simulink model "UberSpurs"  (R2015b)
settings: Solver=VariableStepAuto  StartTime=0.0  StopTime=10000  RelTol=1e-3
(part 2 of 4)

== system UberSpurs/spur1WorkCell/route2Channel12 ==
  serverAvailable : Inport
  Constant : Constant  Value=12
  Get Attribute : GetAttribute  AttributeName=Channel  EvaluatedDefaultAttributeValue={ []}
      settings: OutputPortMap=o1
  RoutingControlBehavior : Stateflow chart  TreatAsAtomicUnit=on
  Single Server1 : SingleServer  ServiceTime=0
  route2Channel1 : OutputSwitch  NumberOutputPorts=2  SwitchingCriterion=From signal port p  InitialConditionsOpt=on
  toChannel : PMIOPort  Port=1  Side=Right
  fromMHS : PMIOPort  Port=2  Side=Left
  toMHS : PMIOPort  Port=3  Side=Right
  wires:
  RoutingControlBehavior/1(route) -> route2Channel1/1
  Constant/1 -> RoutingControlBehavior/2(channel)
  Get Attribute/1 -> RoutingControlBehavior/1(entityChannel)
  serverAvailable/1 -> RoutingControlBehavior/3(serverAvailable)
  connections:
  route2Channel1/RConn2 -- toMHS/RConn1
  Get Attribute/RConn1 -- Single Server1/LConn1
  fromMHS/RConn1 -- Get Attribute/LConn1
  toChannel/RConn1 -- route2Channel1/RConn1
  Single Server1/RConn1 -- route2Channel1/LConn1

== system UberSpurs/spur1WorkCell/route2Channel13 ==
  serverAvailable : Inport
  Constant : Constant  Value=13
  Get Attribute : GetAttribute  AttributeName=Channel  EvaluatedDefaultAttributeValue={ []}
      settings: OutputPortMap=o1
  RoutingControlBehavior : Stateflow chart  TreatAsAtomicUnit=on
  Single Server1 : SingleServer  ServiceTime=0
  route2Channel1 : OutputSwitch  NumberOutputPorts=2  SwitchingCriterion=From signal port p  InitialConditionsOpt=on
  toChannel : PMIOPort  Port=1  Side=Right
  fromMHS : PMIOPort  Port=2  Side=Left
  toMHS : PMIOPort  Port=3  Side=Right
  wires:
  RoutingControlBehavior/1(route) -> route2Channel1/1
  Constant/1 -> RoutingControlBehavior/2(channel)
  Get Attribute/1 -> RoutingControlBehavior/1(entityChannel)
  serverAvailable/1 -> RoutingControlBehavior/3(serverAvailable)
  connections:
  route2Channel1/RConn2 -- toMHS/RConn1
  Get Attribute/RConn1 -- Single Server1/LConn1
  fromMHS/RConn1 -- Get Attribute/LConn1
  toChannel/RConn1 -- route2Channel1/RConn1
  Single Server1/RConn1 -- route2Channel1/LConn1

== system UberSpurs/spur1WorkCell/route2Channel14 ==
  serverAvailable : Inport
  Constant : Constant  Value=14
  Get Attribute : GetAttribute  AttributeName=Channel  EvaluatedDefaultAttributeValue={ []}
      settings: OutputPortMap=o1
  RoutingControlBehavior : Stateflow chart  TreatAsAtomicUnit=on
  Single Server1 : SingleServer  ServiceTime=0
  route2Channel1 : OutputSwitch  NumberOutputPorts=2  SwitchingCriterion=From signal port p  InitialConditionsOpt=on
  toChannel : PMIOPort  Port=1  Side=Right
  fromMHS : PMIOPort  Port=2  Side=Left
  toMHS : PMIOPort  Port=3  Side=Right
  wires:
  RoutingControlBehavior/1(route) -> route2Channel1/1
  Constant/1 -> RoutingControlBehavior/2(channel)
  Get Attribute/1 -> RoutingControlBehavior/1(entityChannel)
  serverAvailable/1 -> RoutingControlBehavior/3(serverAvailable)
  connections:
  route2Channel1/RConn2 -- toMHS/RConn1
  Get Attribute/RConn1 -- Single Server1/LConn1
  fromMHS/RConn1 -- Get Attribute/LConn1
  toChannel/RConn1 -- route2Channel1/RConn1
  Single Server1/RConn1 -- route2Channel1/LConn1

== system UberSpurs/spur1WorkCell/route2Channel15 ==
  serverAvailable : Inport
  Constant : Constant  Value=15
  Get Attribute : GetAttribute  AttributeName=Channel  EvaluatedDefaultAttributeValue={ []}
      settings: OutputPortMap=o1
  RoutingControlBehavior : Stateflow chart  TreatAsAtomicUnit=on
  Single Server1 : SingleServer  ServiceTime=0
  route2Channel1 : OutputSwitch  NumberOutputPorts=2  SwitchingCriterion=From signal port p  InitialConditionsOpt=on
  toChannel : PMIOPort  Port=1  Side=Right
  fromMHS : PMIOPort  Port=2  Side=Left
  toMHS : PMIOPort  Port=3  Side=Right
  wires:
  RoutingControlBehavior/1(route) -> route2Channel1/1
  Constant/1 -> RoutingControlBehavior/2(channel)
  Get Attribute/1 -> RoutingControlBehavior/1(entityChannel)
  serverAvailable/1 -> RoutingControlBehavior/3(serverAvailable)
  connections:
  route2Channel1/RConn2 -- toMHS/RConn1
  Get Attribute/RConn1 -- Single Server1/LConn1
  fromMHS/RConn1 -- Get Attribute/LConn1
  toChannel/RConn1 -- route2Channel1/RConn1
  Single Server1/RConn1 -- route2Channel1/LConn1

== system UberSpurs/spur1WorkCell/route2Channel16 ==
  serverAvailable : Inport
  Constant : Constant  Value=16
  Get Attribute : GetAttribute  AttributeName=Channel  EvaluatedDefaultAttributeValue={ []}
      settings: OutputPortMap=o1
  RoutingControlBehavior : Stateflow chart  TreatAsAtomicUnit=on
  Single Server1 : SingleServer  ServiceTime=0
  route2Channel1 : OutputSwitch  NumberOutputPorts=2  SwitchingCriterion=From signal port p  InitialConditionsOpt=on
  toChannel : PMIOPort  Port=1  Side=Right
  fromMHS : PMIOPort  Port=2  Side=Left
  toMHS : PMIOPort  Port=3  Side=Right
  wires:
  RoutingControlBehavior/1(route) -> route2Channel1/1
  Constant/1 -> RoutingControlBehavior/2(channel)
  Get Attribute/1 -> RoutingControlBehavior/1(entityChannel)
  serverAvailable/1 -> RoutingControlBehavior/3(serverAvailable)
  connections:
  route2Channel1/RConn2 -- toMHS/RConn1
  Get Attribute/RConn1 -- Single Server1/LConn1
  fromMHS/RConn1 -- Get Attribute/LConn1
  toChannel/RConn1 -- route2Channel1/RConn1
  Single Server1/RConn1 -- route2Channel1/LConn1

== system UberSpurs/spur1WorkCell/route2Channel17 ==
  serverAvailable : Inport
  Constant : Constant  Value=17
  Get Attribute : GetAttribute  AttributeName=Channel  EvaluatedDefaultAttributeValue={ []}
      settings: OutputPortMap=o1
  RoutingControlBehavior : Stateflow chart  TreatAsAtomicUnit=on
  Single Server1 : SingleServer  ServiceTime=0
  route2Channel1 : OutputSwitch  NumberOutputPorts=2  SwitchingCriterion=From signal port p  InitialConditionsOpt=on
  toChannel : PMIOPort  Port=1  Side=Right
  fromMHS : PMIOPort  Port=2  Side=Left
  toMHS : PMIOPort  Port=3  Side=Right
  wires:
  RoutingControlBehavior/1(route) -> route2Channel1/1
  Constant/1 -> RoutingControlBehavior/2(channel)
  Get Attribute/1 -> RoutingControlBehavior/1(entityChannel)
  serverAvailable/1 -> RoutingControlBehavior/3(serverAvailable)
  connections:
  route2Channel1/RConn2 -- toMHS/RConn1
  Get Attribute/RConn1 -- Single Server1/LConn1
  fromMHS/RConn1 -- Get Attribute/LConn1
  toChannel/RConn1 -- route2Channel1/RConn1
  Single Server1/RConn1 -- route2Channel1/LConn1

== system UberSpurs/spur1WorkCell/route2Channel18 ==
  serverAvailable : Inport
  Constant : Constant  Value=18
  Get Attribute : GetAttribute  AttributeName=Channel  EvaluatedDefaultAttributeValue={ []}
      settings: OutputPortMap=o1
  RoutingControlBehavior : Stateflow chart  TreatAsAtomicUnit=on
  Single Server1 : SingleServer  ServiceTime=0
  route2Channel1 : OutputSwitch  NumberOutputPorts=2  SwitchingCriterion=From signal port p  InitialConditionsOpt=on
  toChannel : PMIOPort  Port=1  Side=Right
  fromMHS : PMIOPort  Port=2  Side=Left
  toMHS : PMIOPort  Port=3  Side=Right
  wires:
  RoutingControlBehavior/1(route) -> route2Channel1/1
  Constant/1 -> RoutingControlBehavior/2(channel)
  Get Attribute/1 -> RoutingControlBehavior/1(entityChannel)
  serverAvailable/1 -> RoutingControlBehavior/3(serverAvailable)
  connections:
  route2Channel1/RConn2 -- toMHS/RConn1
  Get Attribute/RConn1 -- Single Server1/LConn1
  fromMHS/RConn1 -- Get Attribute/LConn1
  toChannel/RConn1 -- route2Channel1/RConn1
  Single Server1/RConn1 -- route2Channel1/LConn1

== system UberSpurs/spur1WorkCell/route2Channel2 ==
  serverAvailable : Inport
  Constant : Constant  Value=2
  Get Attribute : GetAttribute  AttributeName=Channel  EvaluatedDefaultAttributeValue={ []}
      settings: OutputPortMap=o1
  RoutingControlBehavior : Stateflow chart  TreatAsAtomicUnit=on
  Single Server1 : SingleServer  ServiceTime=0
  route2Channel1 : OutputSwitch  NumberOutputPorts=2  SwitchingCriterion=From signal port p  InitialConditionsOpt=on
  toChannel : PMIOPort  Port=1  Side=Right
  fromMHS : PMIOPort  Port=2  Side=Left
  toMHS : PMIOPort  Port=3  Side=Right
  wires:
  RoutingControlBehavior/1(route) -> route2Channel1/1
  Constant/1 -> RoutingControlBehavior/2(channel)
  Get Attribute/1 -> RoutingControlBehavior/1(entityChannel)
  serverAvailable/1 -> RoutingControlBehavior/3(serverAvailable)
  connections:
  route2Channel1/RConn2 -- toMHS/RConn1
  Get Attribute/RConn1 -- Single Server1/LConn1
  fromMHS/RConn1 -- Get Attribute/LConn1
  toChannel/RConn1 -- route2Channel1/RConn1
  Single Server1/RConn1 -- route2Channel1/LConn1

== system UberSpurs/spur1WorkCell/route2Channel3 ==
  serverAvailable : Inport
  Constant : Constant  Value=3
  Get Attribute : GetAttribute  AttributeName=Channel  EvaluatedDefaultAttributeValue={ []}
      settings: OutputPortMap=o1
  RoutingControlBehavior : Stateflow chart  TreatAsAtomicUnit=on
  Single Server1 : SingleServer  ServiceTime=0
  route2Channel1 : OutputSwitch  NumberOutputPorts=2  SwitchingCriterion=From signal port p  InitialConditionsOpt=on
  toChannel : PMIOPort  Port=1  Side=Right
  fromMHS : PMIOPort  Port=2  Side=Left
  toMHS : PMIOPort  Port=3  Side=Right
  wires:
  RoutingControlBehavior/1(route) -> route2Channel1/1
  Constant/1 -> RoutingControlBehavior/2(channel)
  Get Attribute/1 -> RoutingControlBehavior/1(entityChannel)
  serverAvailable/1 -> RoutingControlBehavior/3(serverAvailable)
  connections:
  route2Channel1/RConn2 -- toMHS/RConn1
  Get Attribute/RConn1 -- Single Server1/LConn1
  fromMHS/RConn1 -- Get Attribute/LConn1
  toChannel/RConn1 -- route2Channel1/RConn1
  Single Server1/RConn1 -- route2Channel1/LConn1

== system UberSpurs/spur1WorkCell/route2Channel4 ==
  serverAvailable : Inport
  Constant : Constant  Value=4
  Get Attribute : GetAttribute  AttributeName=Channel  EvaluatedDefaultAttributeValue={ []}
      settings: OutputPortMap=o1
  RoutingControlBehavior : Stateflow chart  TreatAsAtomicUnit=on
  Single Server1 : SingleServer  ServiceTime=0
  route2Channel1 : OutputSwitch  NumberOutputPorts=2  SwitchingCriterion=From signal port p  InitialConditionsOpt=on
  toChannel : PMIOPort  Port=1  Side=Right
  fromMHS : PMIOPort  Port=2  Side=Left
  toMHS : PMIOPort  Port=3  Side=Right
  wires:
  RoutingControlBehavior/1(route) -> route2Channel1/1
  Constant/1 -> RoutingControlBehavior/2(channel)
  Get Attribute/1 -> RoutingControlBehavior/1(entityChannel)
  serverAvailable/1 -> RoutingControlBehavior/3(serverAvailable)
  connections:
  route2Channel1/RConn2 -- toMHS/RConn1
  Get Attribute/RConn1 -- Single Server1/LConn1
  fromMHS/RConn1 -- Get Attribute/LConn1
  toChannel/RConn1 -- route2Channel1/RConn1
  Single Server1/RConn1 -- route2Channel1/LConn1

== system UberSpurs/spur1WorkCell/route2Channel5 ==
  serverAvailable : Inport
  Constant : Constant  Value=5
  Get Attribute : GetAttribute  AttributeName=Channel  EvaluatedDefaultAttributeValue={ []}
      settings: OutputPortMap=o1
  RoutingControlBehavior : Stateflow chart  TreatAsAtomicUnit=on
  Single Server1 : SingleServer  ServiceTime=0
  route2Channel1 : OutputSwitch  NumberOutputPorts=2  SwitchingCriterion=From signal port p  InitialConditionsOpt=on
  toChannel : PMIOPort  Port=1  Side=Right
  fromMHS : PMIOPort  Port=2  Side=Left
  toMHS : PMIOPort  Port=3  Side=Right
  wires:
  RoutingControlBehavior/1(route) -> route2Channel1/1
  Constant/1 -> RoutingControlBehavior/2(channel)
  Get Attribute/1 -> RoutingControlBehavior/1(entityChannel)
  serverAvailable/1 -> RoutingControlBehavior/3(serverAvailable)
  connections:
  route2Channel1/RConn2 -- toMHS/RConn1
  Get Attribute/RConn1 -- Single Server1/LConn1
  fromMHS/RConn1 -- Get Attribute/LConn1
  toChannel/RConn1 -- route2Channel1/RConn1
  Single Server1/RConn1 -- route2Channel1/LConn1

== system UberSpurs/spur1WorkCell/route2Channel6 ==
  serverAvailable : Inport
  Constant : Constant  Value=6
  Get Attribute : GetAttribute  AttributeName=Channel  EvaluatedDefaultAttributeValue={ []}
      settings: OutputPortMap=o1
  RoutingControlBehavior : Stateflow chart  TreatAsAtomicUnit=on
  Single Server1 : SingleServer  ServiceTime=0
  route2Channel1 : OutputSwitch  NumberOutputPorts=2  SwitchingCriterion=From signal port p  InitialConditionsOpt=on
  toChannel : PMIOPort  Port=1  Side=Right
  fromMHS : PMIOPort  Port=2  Side=Left
  toMHS : PMIOPort  Port=3  Side=Right
  wires:
  RoutingControlBehavior/1(route) -> route2Channel1/1
  Constant/1 -> RoutingControlBehavior/2(channel)
  Get Attribute/1 -> RoutingControlBehavior/1(entityChannel)
  serverAvailable/1 -> RoutingControlBehavior/3(serverAvailable)
  connections:
  route2Channel1/RConn2 -- toMHS/RConn1
  Get Attribute/RConn1 -- Single Server1/LConn1
  fromMHS/RConn1 -- Get Attribute/LConn1
  toChannel/RConn1 -- route2Channel1/RConn1
  Single Server1/RConn1 -- route2Channel1/LConn1

== system UberSpurs/spur1WorkCell/route2Channel7 ==
  serverAvailable : Inport
  Constant : Constant  Value=7
  Get Attribute : GetAttribute  AttributeName=Channel  EvaluatedDefaultAttributeValue={ []}
      settings: OutputPortMap=o1
  RoutingControlBehavior : Stateflow chart  TreatAsAtomicUnit=on
  Single Server1 : SingleServer  ServiceTime=0
  route2Channel1 : OutputSwitch  NumberOutputPorts=2  SwitchingCriterion=From signal port p  InitialConditionsOpt=on
  toChannel : PMIOPort  Port=1  Side=Right
  fromMHS : PMIOPort  Port=2  Side=Left
  toMHS : PMIOPort  Port=3  Side=Right
  wires:
  RoutingControlBehavior/1(route) -> route2Channel1/1
  Constant/1 -> RoutingControlBehavior/2(channel)
  Get Attribute/1 -> RoutingControlBehavior/1(entityChannel)
  serverAvailable/1 -> RoutingControlBehavior/3(serverAvailable)
  connections:
  route2Channel1/RConn2 -- toMHS/RConn1
  Get Attribute/RConn1 -- Single Server1/LConn1
  fromMHS/RConn1 -- Get Attribute/LConn1
  toChannel/RConn1 -- route2Channel1/RConn1
  Single Server1/RConn1 -- route2Channel1/LConn1

== system UberSpurs/spur1WorkCell/route2Channel8 ==
  serverAvailable : Inport
  Constant : Constant  Value=8
  Get Attribute : GetAttribute  AttributeName=Channel  EvaluatedDefaultAttributeValue={ []}
      settings: OutputPortMap=o1
  RoutingControlBehavior : Stateflow chart  TreatAsAtomicUnit=on
  Single Server1 : SingleServer  ServiceTime=0
  route2Channel1 : OutputSwitch  NumberOutputPorts=2  SwitchingCriterion=From signal port p  InitialConditionsOpt=on
  toChannel : PMIOPort  Port=1  Side=Right
  fromMHS : PMIOPort  Port=2  Side=Left
  toMHS : PMIOPort  Port=3  Side=Right
  wires:
  RoutingControlBehavior/1(route) -> route2Channel1/1
  Constant/1 -> RoutingControlBehavior/2(channel)
  Get Attribute/1 -> RoutingControlBehavior/1(entityChannel)
  serverAvailable/1 -> RoutingControlBehavior/3(serverAvailable)
  connections:
  route2Channel1/RConn2 -- toMHS/RConn1
  Get Attribute/RConn1 -- Single Server1/LConn1
  fromMHS/RConn1 -- Get Attribute/LConn1
  toChannel/RConn1 -- route2Channel1/RConn1
  Single Server1/RConn1 -- route2Channel1/LConn1

== system UberSpurs/spur1WorkCell/route2Channel9 ==
  serverAvailable : Inport
  Constant : Constant  Value=9
  Get Attribute : GetAttribute  AttributeName=Channel  EvaluatedDefaultAttributeValue={ []}
      settings: OutputPortMap=o1
  RoutingControlBehavior : Stateflow chart  TreatAsAtomicUnit=on
  Single Server1 : SingleServer  ServiceTime=0
  route2Channel1 : OutputSwitch  NumberOutputPorts=2  SwitchingCriterion=From signal port p  InitialConditionsOpt=on
  toChannel : PMIOPort  Port=1  Side=Right
  fromMHS : PMIOPort  Port=2  Side=Left
  toMHS : PMIOPort  Port=3  Side=Right
  wires:
  RoutingControlBehavior/1(route) -> route2Channel1/1
  Constant/1 -> RoutingControlBehavior/2(channel)
  Get Attribute/1 -> RoutingControlBehavior/1(entityChannel)
  serverAvailable/1 -> RoutingControlBehavior/3(serverAvailable)
  connections:
  route2Channel1/RConn2 -- toMHS/RConn1
  Get Attribute/RConn1 -- Single Server1/LConn1
  fromMHS/RConn1 -- Get Attribute/LConn1
  toChannel/RConn1 -- route2Channel1/RConn1
  Single Server1/RConn1 -- route2Channel1/LConn1

== system UberSpurs/spur1WorkCell/route2recirculate ==
  verifyQueueLength : Inport
  Chart : Stateflow chart  TreatAsAtomicUnit=on
  Get Attribute : GetAttribute  AttributeName=FillTime  EvaluatedDefaultAttributeValue={ []}
      settings: OutputPortMap=o1
  Single Server1 : SingleServer  ServiceTime=0
  route2recirculate : OutputSwitch  NumberOutputPorts=2  SwitchingCriterion=From signal port p  InitialConditionsOpt=on  StatNumberDeparted=on  StatLastDeparturePort=on
      settings: OutputPortMap=o0,o3
  recirculate : PMIOPort  Port=1  Side=Right
  fromMHS : PMIOPort  Port=2  Side=Left
  toverify : PMIOPort  Port=3  Side=Right
  wires:
  Chart/1(route) -> route2recirculate/1
  Get Attribute/1 -> Chart/1(FillTime)
  route2recirculate/1 -> ?
  route2recirculate/2 -> ?
  verifyQueueLength/1 -> Chart/2(verifyQueue)
  connections:
  Get Attribute/RConn1 -- Single Server1/LConn1
  fromMHS/RConn1 -- Get Attribute/LConn1
  Single Server1/RConn1 -- route2recirculate/LConn1
  route2recirculate/RConn2 -- toverify/RConn1
  route2recirculate/RConn1 -- recirculate/RConn1

== system UberSpurs/spur1WorkCell/verifyWorkstation ==
  Clock : Clock
  Set Attribute1 : SetAttribute  AttributeName=VerifyTime  AttributeFrom=Signal port  EvaluatedAttributeValue={ []}
  Timed to Event Sigal : TimedToEventSignal
  VerifyQueue : FIFOQueue  Capacity=12  StatNumberInBlock=on
      settings: OutputPortMap=o1
  VerifyServer : SingleServer  ServiceTimeFrom=Signal port t  ServiceTime=1.55
  processTime : EventBasedRandomNumber  Distribution=Arbitrary discrete  valueVecDisc=[0 1.55]  probVecDisc=[0 1]  Seed=19165
  vialOUT : PMIOPort  Port=1  Side=Left
  vialIN : PMIOPort  Port=2  Side=Right
  queueLength : Outport
  wires:
  processTime/1 -> VerifyServer/1
  Clock/1 -> Timed to Event Sigal/1
  Timed to Event Sigal/1 -> Set Attribute1/1
  VerifyQueue/1 -> queueLength/1
  connections:
  Set Attribute1/RConn1 -- vialOUT/RConn1
  VerifyQueue/RConn1 -- VerifyServer/LConn1
  VerifyQueue/LConn1 -- vialIN/RConn1
  Set Attribute1/LConn1 -- VerifyServer/RConn1

== system UberSpurs/spur2WorkCell/fillChannel1 ==
  Clock : Clock
  Set Attribute : SetAttribute  AttributeName=FillTime  AttributeFrom=Signal port  EvaluatedAttributeValue={ []}
  Timed to Event Signal : TimedToEventSignal
  fillQueue : FIFOQueue  Capacity=1
  fillServer : SingleServer  ServiceTimeFrom=Signal port t  ServiceTime=20  StatNumberInBlock=on
      settings: OutputPortMap=o1
  processTime : EventBasedRandomNumber  Distribution=Gaussian (normal)  meanNorm=25  stdNorm=2.5  Seed=22382
  vialIN : PMIOPort  Port=1  Side=Left
  vialOut : PMIOPort  Port=2  Side=Right
  serverAvailable : Outport
  wires:
  processTime/1 -> fillServer/1
  Clock/1 -> Timed to Event Signal/1
  Timed to Event Signal/1 -> Set Attribute/1
  fillServer/1 -> serverAvailable/1
  connections:
  fillQueue/RConn1 -- fillServer/LConn1
  fillQueue/LConn1 -- vialIN/RConn1
  fillServer/RConn1 -- Set Attribute/LConn1
  Set Attribute/RConn1 -- vialOut/RConn1

== system UberSpurs/spur2WorkCell/fillChannel10 ==
  Clock : Clock
  Set Attribute : SetAttribute  AttributeName=FillTime  AttributeFrom=Signal port  EvaluatedAttributeValue={ []}
  Timed to Event Signal : TimedToEventSignal
  fillQueue : FIFOQueue  Capacity=1
  fillServer : SingleServer  ServiceTimeFrom=Signal port t  ServiceTime=20  StatNumberInBlock=on
      settings: OutputPortMap=o1
  processTime : EventBasedRandomNumber  Distribution=Gaussian (normal)  meanNorm=25  stdNorm=2.5  Seed=25599
  vialIN : PMIOPort  Port=1  Side=Left
  vialOut : PMIOPort  Port=2  Side=Right
  serverAvailable : Outport
  wires:
  processTime/1 -> fillServer/1
  Clock/1 -> Timed to Event Signal/1
  Timed to Event Signal/1 -> Set Attribute/1
  fillServer/1 -> serverAvailable/1
  connections:
  fillQueue/RConn1 -- fillServer/LConn1
  fillQueue/LConn1 -- vialIN/RConn1
  fillServer/RConn1 -- Set Attribute/LConn1
  Set Attribute/RConn1 -- vialOut/RConn1

== system UberSpurs/spur2WorkCell/fillChannel11 ==
  Clock : Clock
  Set Attribute : SetAttribute  AttributeName=FillTime  AttributeFrom=Signal port  EvaluatedAttributeValue={ []}
  Timed to Event Signal : TimedToEventSignal
  fillQueue : FIFOQueue  Capacity=1
  fillServer : SingleServer  ServiceTimeFrom=Signal port t  ServiceTime=20  StatNumberInBlock=on
      settings: OutputPortMap=o1
  processTime : EventBasedRandomNumber  Distribution=Gaussian (normal)  meanNorm=25  stdNorm=2.5  Seed=28816
  vialIN : PMIOPort  Port=1  Side=Left
  vialOut : PMIOPort  Port=2  Side=Right
  serverAvailable : Outport
  wires:
  processTime/1 -> fillServer/1
  Clock/1 -> Timed to Event Signal/1
  Timed to Event Signal/1 -> Set Attribute/1
  fillServer/1 -> serverAvailable/1
  connections:
  fillQueue/RConn1 -- fillServer/LConn1
  fillQueue/LConn1 -- vialIN/RConn1
  fillServer/RConn1 -- Set Attribute/LConn1
  Set Attribute/RConn1 -- vialOut/RConn1

== system UberSpurs/spur2WorkCell/fillChannel12 ==
  Clock : Clock
  Set Attribute : SetAttribute  AttributeName=FillTime  AttributeFrom=Signal port  EvaluatedAttributeValue={ []}
  Timed to Event Signal : TimedToEventSignal
  fillQueue : FIFOQueue  Capacity=1
  fillServer : SingleServer  ServiceTimeFrom=Signal port t  ServiceTime=20  StatNumberInBlock=on
      settings: OutputPortMap=o1
  processTime : EventBasedRandomNumber  Distribution=Gaussian (normal)  meanNorm=25  stdNorm=2.5  Seed=32033
  vialIN : PMIOPort  Port=1  Side=Left
  vialOut : PMIOPort  Port=2  Side=Right
  serverAvailable : Outport
  wires:
  processTime/1 -> fillServer/1
  Clock/1 -> Timed to Event Signal/1
  Timed to Event Signal/1 -> Set Attribute/1
  fillServer/1 -> serverAvailable/1
  connections:
  fillQueue/RConn1 -- fillServer/LConn1
  fillQueue/LConn1 -- vialIN/RConn1
  fillServer/RConn1 -- Set Attribute/LConn1
  Set Attribute/RConn1 -- vialOut/RConn1

== system UberSpurs/spur2WorkCell/fillChannel13 ==
  Clock : Clock
  Set Attribute : SetAttribute  AttributeName=FillTime  AttributeFrom=Signal port  EvaluatedAttributeValue={ []}
  Timed to Event Signal : TimedToEventSignal
  fillQueue : FIFOQueue  Capacity=1
  fillServer : SingleServer  ServiceTimeFrom=Signal port t  ServiceTime=20  StatNumberInBlock=on
      settings: OutputPortMap=o1
  processTime : EventBasedRandomNumber  Distribution=Gaussian (normal)  meanNorm=25  stdNorm=2.5  Seed=35250
  vialIN : PMIOPort  Port=1  Side=Left
  vialOut : PMIOPort  Port=2  Side=Right
  serverAvailable : Outport
  wires:
  processTime/1 -> fillServer/1
  Clock/1 -> Timed to Event Signal/1
  Timed to Event Signal/1 -> Set Attribute/1
  fillServer/1 -> serverAvailable/1
  connections:
  fillQueue/RConn1 -- fillServer/LConn1
  fillQueue/LConn1 -- vialIN/RConn1
  fillServer/RConn1 -- Set Attribute/LConn1
  Set Attribute/RConn1 -- vialOut/RConn1

== system UberSpurs/spur2WorkCell/fillChannel14 ==
  Clock : Clock
  Set Attribute : SetAttribute  AttributeName=FillTime  AttributeFrom=Signal port  EvaluatedAttributeValue={ []}
  Timed to Event Signal : TimedToEventSignal
  fillQueue : FIFOQueue  Capacity=1
  fillServer : SingleServer  ServiceTimeFrom=Signal port t  ServiceTime=20  StatNumberInBlock=on
      settings: OutputPortMap=o1
  processTime : EventBasedRandomNumber  Distribution=Gaussian (normal)  meanNorm=25  stdNorm=2.5  Seed=38467
  vialIN : PMIOPort  Port=1  Side=Left
  vialOut : PMIOPort  Port=2  Side=Right
  serverAvailable : Outport
  wires:
  processTime/1 -> fillServer/1
  Clock/1 -> Timed to Event Signal/1
  Timed to Event Signal/1 -> Set Attribute/1
  fillServer/1 -> serverAvailable/1
  connections:
  fillQueue/RConn1 -- fillServer/LConn1
  fillQueue/LConn1 -- vialIN/RConn1
  fillServer/RConn1 -- Set Attribute/LConn1
  Set Attribute/RConn1 -- vialOut/RConn1

== system UberSpurs/spur2WorkCell/fillChannel15 ==
  Clock : Clock
  Set Attribute : SetAttribute  AttributeName=FillTime  AttributeFrom=Signal port  EvaluatedAttributeValue={ []}
  Timed to Event Signal : TimedToEventSignal
  fillQueue : FIFOQueue  Capacity=1
  fillServer : SingleServer  ServiceTimeFrom=Signal port t  ServiceTime=20  StatNumberInBlock=on
      settings: OutputPortMap=o1
  processTime : EventBasedRandomNumber  Distribution=Gaussian (normal)  meanNorm=25  stdNorm=2.5  Seed=41684
  vialIN : PMIOPort  Port=1  Side=Left
  vialOut : PMIOPort  Port=2  Side=Right
  serverAvailable : Outport
  wires:
  processTime/1 -> fillServer/1
  Clock/1 -> Timed to Event Signal/1
  Timed to Event Signal/1 -> Set Attribute/1
  fillServer/1 -> serverAvailable/1
  connections:
  fillQueue/RConn1 -- fillServer/LConn1
  fillQueue/LConn1 -- vialIN/RConn1
  fillServer/RConn1 -- Set Attribute/LConn1
  Set Attribute/RConn1 -- vialOut/RConn1

== system UberSpurs/spur2WorkCell/fillChannel16 ==
  Clock : Clock
  Set Attribute : SetAttribute  AttributeName=FillTime  AttributeFrom=Signal port  EvaluatedAttributeValue={ []}
  Timed to Event Signal : TimedToEventSignal
  fillQueue : FIFOQueue  Capacity=1
  fillServer : SingleServer  ServiceTimeFrom=Signal port t  ServiceTime=20  StatNumberInBlock=on
      settings: OutputPortMap=o1
  processTime : EventBasedRandomNumber  Distribution=Gaussian (normal)  meanNorm=25  stdNorm=2.5  Seed=44901
  vialIN : PMIOPort  Port=1  Side=Left
  vialOut : PMIOPort  Port=2  Side=Right
  serverAvailable : Outport
  wires:
  processTime/1 -> fillServer/1
  Clock/1 -> Timed to Event Signal/1
  Timed to Event Signal/1 -> Set Attribute/1
  fillServer/1 -> serverAvailable/1
  connections:
  fillQueue/RConn1 -- fillServer/LConn1
  fillQueue/LConn1 -- vialIN/RConn1
  fillServer/RConn1 -- Set Attribute/LConn1
  Set Attribute/RConn1 -- vialOut/RConn1

== system UberSpurs/spur2WorkCell/fillChannel17 ==
  Clock : Clock
  Set Attribute : SetAttribute  AttributeName=FillTime  AttributeFrom=Signal port  EvaluatedAttributeValue={ []}
  Timed to Event Signal : TimedToEventSignal
  fillQueue : FIFOQueue  Capacity=1
  fillServer : SingleServer  ServiceTimeFrom=Signal port t  ServiceTime=20  StatNumberInBlock=on
      settings: OutputPortMap=o1
  processTime : EventBasedRandomNumber  Distribution=Gaussian (normal)  meanNorm=25  stdNorm=2.5  Seed=48118
  vialIN : PMIOPort  Port=1  Side=Left
  vialOut : PMIOPort  Port=2  Side=Right
  serverAvailable : Outport
  wires:
  processTime/1 -> fillServer/1
  Clock/1 -> Timed to Event Signal/1
  Timed to Event Signal/1 -> Set Attribute/1
  fillServer/1 -> serverAvailable/1
  connections:
  fillQueue/RConn1 -- fillServer/LConn1
  fillQueue/LConn1 -- vialIN/RConn1
  fillServer/RConn1 -- Set Attribute/LConn1
  Set Attribute/RConn1 -- vialOut/RConn1

== system UberSpurs/spur2WorkCell/fillChannel18 ==
  Clock : Clock
  Set Attribute : SetAttribute  AttributeName=FillTime  AttributeFrom=Signal port  EvaluatedAttributeValue={ []}
  Timed to Event Signal : TimedToEventSignal
  fillQueue : FIFOQueue  Capacity=1
  fillServer : SingleServer  ServiceTimeFrom=Signal port t  ServiceTime=20  StatNumberInBlock=on
      settings: OutputPortMap=o1
  processTime : EventBasedRandomNumber  Distribution=Gaussian (normal)  meanNorm=25  stdNorm=2.5  Seed=51335
  vialIN : PMIOPort  Port=1  Side=Left
  vialOut : PMIOPort  Port=2  Side=Right
  serverAvailable : Outport
  wires:
  processTime/1 -> fillServer/1
  Clock/1 -> Timed to Event Signal/1
  Timed to Event Signal/1 -> Set Attribute/1
  fillServer/1 -> serverAvailable/1
  connections:
  fillQueue/RConn1 -- fillServer/LConn1
  fillQueue/LConn1 -- vialIN/RConn1
  fillServer/RConn1 -- Set Attribute/LConn1
  Set Attribute/RConn1 -- vialOut/RConn1

== system UberSpurs/spur2WorkCell/fillChannel2 ==
  Clock : Clock
  Set Attribute : SetAttribute  AttributeName=FillTime  AttributeFrom=Signal port  EvaluatedAttributeValue={ []}
  Timed to Event Signal : TimedToEventSignal
  fillQueue : FIFOQueue  Capacity=1
  fillServer : SingleServer  ServiceTimeFrom=Signal port t  ServiceTime=20  StatNumberInBlock=on
      settings: OutputPortMap=o1
  processTime : EventBasedRandomNumber  Distribution=Gaussian (normal)  meanNorm=25  stdNorm=2.5  Seed=54552
  vialIN : PMIOPort  Port=1  Side=Left
  vialOut : PMIOPort  Port=2  Side=Right
  serverAvailable : Outport
  wires:
  processTime/1 -> fillServer/1
  Clock/1 -> Timed to Event Signal/1
  Timed to Event Signal/1 -> Set Attribute/1
  fillServer/1 -> serverAvailable/1
  connections:
  fillQueue/RConn1 -- fillServer/LConn1
  fillQueue/LConn1 -- vialIN/RConn1
  fillServer/RConn1 -- Set Attribute/LConn1
  Set Attribute/RConn1 -- vialOut/RConn1

== system UberSpurs/spur2WorkCell/fillChannel3 ==
  Clock : Clock
  Set Attribute : SetAttribute  AttributeName=FillTime  AttributeFrom=Signal port  EvaluatedAttributeValue={ []}
  Timed to Event Signal : TimedToEventSignal
  fillQueue : FIFOQueue  Capacity=1
  fillServer : SingleServer  ServiceTimeFrom=Signal port t  ServiceTime=20  StatNumberInBlock=on
      settings: OutputPortMap=o1
  processTime : EventBasedRandomNumber  Distribution=Gaussian (normal)  meanNorm=25  stdNorm=2.5  Seed=57769
  vialIN : PMIOPort  Port=1  Side=Left
  vialOut : PMIOPort  Port=2  Side=Right
  serverAvailable : Outport
  wires:
  processTime/1 -> fillServer/1
  Clock/1 -> Timed to Event Signal/1
  Timed to Event Signal/1 -> Set Attribute/1
  fillServer/1 -> serverAvailable/1
  connections:
  fillQueue/RConn1 -- fillServer/LConn1
  fillQueue/LConn1 -- vialIN/RConn1
  fillServer/RConn1 -- Set Attribute/LConn1
  Set Attribute/RConn1 -- vialOut/RConn1

== system UberSpurs/spur2WorkCell/fillChannel4 ==
  Clock : Clock
  Set Attribute : SetAttribute  AttributeName=FillTime  AttributeFrom=Signal port  EvaluatedAttributeValue={ []}
  Timed to Event Signal : TimedToEventSignal
  fillQueue : FIFOQueue  Capacity=1
  fillServer : SingleServer  ServiceTimeFrom=Signal port t  ServiceTime=20  StatNumberInBlock=on
      settings: OutputPortMap=o1
  processTime : EventBasedRandomNumber  Distribution=Gaussian (normal)  meanNorm=25  stdNorm=2.5  Seed=60986
  vialIN : PMIOPort  Port=1  Side=Left
  vialOut : PMIOPort  Port=2  Side=Right
  serverAvailable : Outport
  wires:
  processTime/1 -> fillServer/1
  Clock/1 -> Timed to Event Signal/1
  Timed to Event Signal/1 -> Set Attribute/1
  fillServer/1 -> serverAvailable/1
  connections:
  fillQueue/RConn1 -- fillServer/LConn1
  fillQueue/LConn1 -- vialIN/RConn1
  fillServer/RConn1 -- Set Attribute/LConn1
  Set Attribute/RConn1 -- vialOut/RConn1

== system UberSpurs/spur2WorkCell/fillChannel5 ==
  Clock : Clock
  Set Attribute : SetAttribute  AttributeName=FillTime  AttributeFrom=Signal port  EvaluatedAttributeValue={ []}
  Timed to Event Signal : TimedToEventSignal
  fillQueue : FIFOQueue  Capacity=1
  fillServer : SingleServer  ServiceTimeFrom=Signal port t  ServiceTime=20  StatNumberInBlock=on
      settings: OutputPortMap=o1
  processTime : EventBasedRandomNumber  Distribution=Gaussian (normal)  meanNorm=25  stdNorm=2.5  Seed=64203
  vialIN : PMIOPort  Port=1  Side=Left
  vialOut : PMIOPort  Port=2  Side=Right
  serverAvailable : Outport
  wires:
  processTime/1 -> fillServer/1
  Clock/1 -> Timed to Event Signal/1
  Timed to Event Signal/1 -> Set Attribute/1
  fillServer/1 -> serverAvailable/1
  connections:
  fillQueue/RConn1 -- fillServer/LConn1
  fillQueue/LConn1 -- vialIN/RConn1
  fillServer/RConn1 -- Set Attribute/LConn1
  Set Attribute/RConn1 -- vialOut/RConn1

== system UberSpurs/spur2WorkCell/fillChannel6 ==
  Clock : Clock
  Set Attribute : SetAttribute  AttributeName=FillTime  AttributeFrom=Signal port  EvaluatedAttributeValue={ []}
  Timed to Event Signal : TimedToEventSignal
  fillQueue : FIFOQueue  Capacity=1
  fillServer : SingleServer  ServiceTimeFrom=Signal port t  ServiceTime=20  StatNumberInBlock=on
      settings: OutputPortMap=o1
  processTime : EventBasedRandomNumber  Distribution=Gaussian (normal)  meanNorm=25  stdNorm=2.5  Seed=1884
  vialIN : PMIOPort  Port=1  Side=Left
  vialOut : PMIOPort  Port=2  Side=Right
  serverAvailable : Outport
  wires:
  processTime/1 -> fillServer/1
  Clock/1 -> Timed to Event Signal/1
  Timed to Event Signal/1 -> Set Attribute/1
  fillServer/1 -> serverAvailable/1
  connections:
  fillQueue/RConn1 -- fillServer/LConn1
  fillQueue/LConn1 -- vialIN/RConn1
  fillServer/RConn1 -- Set Attribute/LConn1
  Set Attribute/RConn1 -- vialOut/RConn1

== system UberSpurs/spur2WorkCell/fillChannel7 ==
  Clock : Clock
  Set Attribute : SetAttribute  AttributeName=FillTime  AttributeFrom=Signal port  EvaluatedAttributeValue={ []}
  Timed to Event Signal : TimedToEventSignal
  fillQueue : FIFOQueue  Capacity=1
  fillServer : SingleServer  ServiceTimeFrom=Signal port t  ServiceTime=20  StatNumberInBlock=on
      settings: OutputPortMap=o1
  processTime : EventBasedRandomNumber  Distribution=Gaussian (normal)  meanNorm=25  stdNorm=2.5  Seed=5101
  vialIN : PMIOPort  Port=1  Side=Left
  vialOut : PMIOPort  Port=2  Side=Right
  serverAvailable : Outport
  wires:
  processTime/1 -> fillServer/1
  Clock/1 -> Timed to Event Signal/1
  Timed to Event Signal/1 -> Set Attribute/1
  fillServer/1 -> serverAvailable/1
  connections:
  fillQueue/RConn1 -- fillServer/LConn1
  fillQueue/LConn1 -- vialIN/RConn1
  fillServer/RConn1 -- Set Attribute/LConn1
  Set Attribute/RConn1 -- vialOut/RConn1

== system UberSpurs/spur2WorkCell/fillChannel8 ==
  Clock : Clock
  Set Attribute : SetAttribute  AttributeName=FillTime  AttributeFrom=Signal port  EvaluatedAttributeValue={ []}
  Timed to Event Signal : TimedToEventSignal
  fillQueue : FIFOQueue  Capacity=1
  fillServer : SingleServer  ServiceTimeFrom=Signal port t  ServiceTime=20  StatNumberInBlock=on
      settings: OutputPortMap=o1
  processTime : EventBasedRandomNumber  Distribution=Gaussian (normal)  meanNorm=25  stdNorm=2.5  Seed=8318
  vialIN : PMIOPort  Port=1  Side=Left
  vialOut : PMIOPort  Port=2  Side=Right
  serverAvailable : Outport
  wires:
  processTime/1 -> fillServer/1
  Clock/1 -> Timed to Event Signal/1
  Timed to Event Signal/1 -> Set Attribute/1
  fillServer/1 -> serverAvailable/1
  connections:
  fillQueue/RConn1 -- fillServer/LConn1
  fillQueue/LConn1 -- vialIN/RConn1
  fillServer/RConn1 -- Set Attribute/LConn1
  Set Attribute/RConn1 -- vialOut/RConn1

== system UberSpurs/spur2WorkCell/fillChannel9 ==
  Clock : Clock
  Set Attribute : SetAttribute  AttributeName=FillTime  AttributeFrom=Signal port  EvaluatedAttributeValue={ []}
  Timed to Event Signal : TimedToEventSignal
  fillQueue : FIFOQueue  Capacity=1
  fillServer : SingleServer  ServiceTimeFrom=Signal port t  ServiceTime=20  StatNumberInBlock=on
      settings: OutputPortMap=o1
  processTime : EventBasedRandomNumber  Distribution=Gaussian (normal)  meanNorm=25  stdNorm=2.5  Seed=11535
  vialIN : PMIOPort  Port=1  Side=Left
  vialOut : PMIOPort  Port=2  Side=Right
  serverAvailable : Outport
  wires:
  processTime/1 -> fillServer/1
  Clock/1 -> Timed to Event Signal/1
  Timed to Event Signal/1 -> Set Attribute/1
  fillServer/1 -> serverAvailable/1
  connections:
  fillQueue/RConn1 -- fillServer/LConn1
  fillQueue/LConn1 -- vialIN/RConn1
  fillServer/RConn1 -- Set Attribute/LConn1
  Set Attribute/RConn1 -- vialOut/RConn1

== system UberSpurs/spur2WorkCell/route2Channel1 ==
  serverAvailable : Inport
  Constant : Constant
  Get Attribute : GetAttribute  AttributeName=Channel  EvaluatedDefaultAttributeValue={ []}
      settings: OutputPortMap=o1
  RoutingControlActuator : OutputSwitch  NumberOutputPorts=2  SwitchingCriterion=From signal port p  InitialConditionsOpt=on
  RoutingControlBehavior : Stateflow chart  TreatAsAtomicUnit=on
  Single Server1 : SingleServer  ServiceTime=0
  toChannel : PMIOPort  Port=1  Side=Right
  fromMHS : PMIOPort  Port=2  Side=Left
  toMHS : PMIOPort  Port=3  Side=Right
  wires:
  RoutingControlBehavior/1(route) -> RoutingControlActuator/1
  Constant/1 -> RoutingControlBehavior/2(channel)
  Get Attribute/1 -> RoutingControlBehavior/1(entityChannel)
  serverAvailable/1 -> RoutingControlBehavior/3(serverAvailable)
  connections:
  RoutingControlActuator/RConn2 -- toMHS/RConn1
  Get Attribute/RConn1 -- Single Server1/LConn1
  fromMHS/RConn1 -- Get Attribute/LConn1
  toChannel/RConn1 -- RoutingControlActuator/RConn1
  Single Server1/RConn1 -- RoutingControlActuator/LConn1

== system UberSpurs/spur2WorkCell/route2Channel10 ==
  serverAvailable : Inport
  Constant : Constant  Value=10
  Get Attribute : GetAttribute  AttributeName=Channel  EvaluatedDefaultAttributeValue={ []}
      settings: OutputPortMap=o1
  RoutingControlBehavior : Stateflow chart  TreatAsAtomicUnit=on
  Single Server1 : SingleServer  ServiceTime=0
  route2Channel1 : OutputSwitch  NumberOutputPorts=2  SwitchingCriterion=From signal port p  InitialConditionsOpt=on
  toChannel : PMIOPort  Port=1  Side=Right
  fromMHS : PMIOPort  Port=2  Side=Left
  toMHS : PMIOPort  Port=3  Side=Right
  wires:
  RoutingControlBehavior/1(route) -> route2Channel1/1
  Constant/1 -> RoutingControlBehavior/2(channel)
  Get Attribute/1 -> RoutingControlBehavior/1(entityChannel)
  serverAvailable/1 -> RoutingControlBehavior/3(serverAvailable)
  connections:
  route2Channel1/RConn2 -- toMHS/RConn1
  Get Attribute/RConn1 -- Single Server1/LConn1
  fromMHS/RConn1 -- Get Attribute/LConn1
  toChannel/RConn1 -- route2Channel1/RConn1
  Single Server1/RConn1 -- route2Channel1/LConn1

== system UberSpurs/spur2WorkCell/route2Channel11 ==
  serverAvailable : Inport
  Constant : Constant  Value=11
  Get Attribute : GetAttribute  AttributeName=Channel  EvaluatedDefaultAttributeValue={ []}
      settings: OutputPortMap=o1
  RoutingControlBehavior : Stateflow chart  TreatAsAtomicUnit=on
  Single Server1 : SingleServer  ServiceTime=0
  route2Channel1 : OutputSwitch  NumberOutputPorts=2  SwitchingCriterion=From signal port p  InitialConditionsOpt=on
  toChannel : PMIOPort  Port=1  Side=Right
  fromMHS : PMIOPort  Port=2  Side=Left
  toMHS : PMIOPort  Port=3  Side=Right
  wires:
  RoutingControlBehavior/1(route) -> route2Channel1/1
  Constant/1 -> RoutingControlBehavior/2(channel)
  Get Attribute/1 -> RoutingControlBehavior/1(entityChannel)
  serverAvailable/1 -> RoutingControlBehavior/3(serverAvailable)
  connections:
  route2Channel1/RConn2 -- toMHS/RConn1
  Get Attribute/RConn1 -- Single Server1/LConn1
  fromMHS/RConn1 -- Get Attribute/LConn1
  toChannel/RConn1 -- route2Channel1/RConn1
  Single Server1/RConn1 -- route2Channel1/LConn1

== system UberSpurs/spur2WorkCell/route2Channel12 ==
  serverAvailable : Inport
  Constant : Constant  Value=12
  Get Attribute : GetAttribute  AttributeName=Channel  EvaluatedDefaultAttributeValue={ []}
      settings: OutputPortMap=o1
  RoutingControlBehavior : Stateflow chart  TreatAsAtomicUnit=on
  Single Server1 : SingleServer  ServiceTime=0
  route2Channel1 : OutputSwitch  NumberOutputPorts=2  SwitchingCriterion=From signal port p  InitialConditionsOpt=on
  toChannel : PMIOPort  Port=1  Side=Right
  fromMHS : PMIOPort  Port=2  Side=Left
  toMHS : PMIOPort  Port=3  Side=Right
  wires:
  RoutingControlBehavior/1(route) -> route2Channel1/1
  Constant/1 -> RoutingControlBehavior/2(channel)
  Get Attribute/1 -> RoutingControlBehavior/1(entityChannel)
  serverAvailable/1 -> RoutingControlBehavior/3(serverAvailable)
  connections:
  route2Channel1/RConn2 -- toMHS/RConn1
  Get Attribute/RConn1 -- Single Server1/LConn1
  fromMHS/RConn1 -- Get Attribute/LConn1
  toChannel/RConn1 -- route2Channel1/RConn1
  Single Server1/RConn1 -- route2Channel1/LConn1

== system UberSpurs/spur2WorkCell/route2Channel13 ==
  serverAvailable : Inport
  Constant : Constant  Value=13
  Get Attribute : GetAttribute  AttributeName=Channel  EvaluatedDefaultAttributeValue={ []}
      settings: OutputPortMap=o1
  RoutingControlBehavior : Stateflow chart  TreatAsAtomicUnit=on
  Single Server1 : SingleServer  ServiceTime=0
  route2Channel1 : OutputSwitch  NumberOutputPorts=2  SwitchingCriterion=From signal port p  InitialConditionsOpt=on
  toChannel : PMIOPort  Port=1  Side=Right
  fromMHS : PMIOPort  Port=2  Side=Left
  toMHS : PMIOPort  Port=3  Side=Right
  wires:
  RoutingControlBehavior/1(route) -> route2Channel1/1
  Constant/1 -> RoutingControlBehavior/2(channel)
  Get Attribute/1 -> RoutingControlBehavior/1(entityChannel)
  serverAvailable/1 -> RoutingControlBehavior/3(serverAvailable)
  connections:
  route2Channel1/RConn2 -- toMHS/RConn1
  Get Attribute/RConn1 -- Single Server1/LConn1
  fromMHS/RConn1 -- Get Attribute/LConn1
  toChannel/RConn1 -- route2Channel1/RConn1
  Single Server1/RConn1 -- route2Channel1/LConn1

== system UberSpurs/spur2WorkCell/route2Channel14 ==
  serverAvailable : Inport
  Constant : Constant  Value=14
  Get Attribute : GetAttribute  AttributeName=Channel  EvaluatedDefaultAttributeValue={ []}
      settings: OutputPortMap=o1
  RoutingControlBehavior : Stateflow chart  TreatAsAtomicUnit=on
  Single Server1 : SingleServer  ServiceTime=0
  route2Channel1 : OutputSwitch  NumberOutputPorts=2  SwitchingCriterion=From signal port p  InitialConditionsOpt=on
  toChannel : PMIOPort  Port=1  Side=Right
  fromMHS : PMIOPort  Port=2  Side=Left
  toMHS : PMIOPort  Port=3  Side=Right
  wires:
  RoutingControlBehavior/1(route) -> route2Channel1/1
  Constant/1 -> RoutingControlBehavior/2(channel)
  Get Attribute/1 -> RoutingControlBehavior/1(entityChannel)
  serverAvailable/1 -> RoutingControlBehavior/3(serverAvailable)
  connections:
  route2Channel1/RConn2 -- toMHS/RConn1
  Get Attribute/RConn1 -- Single Server1/LConn1
  fromMHS/RConn1 -- Get Attribute/LConn1
  toChannel/RConn1 -- route2Channel1/RConn1
  Single Server1/RConn1 -- route2Channel1/LConn1

== system UberSpurs/spur2WorkCell/route2Channel15 ==
  serverAvailable : Inport
  Constant : Constant  Value=15
  Get Attribute : GetAttribute  AttributeName=Channel  EvaluatedDefaultAttributeValue={ []}
      settings: OutputPortMap=o1
  RoutingControlBehavior : Stateflow chart  TreatAsAtomicUnit=on
  Single Server1 : SingleServer  ServiceTime=0
  route2Channel1 : OutputSwitch  NumberOutputPorts=2  SwitchingCriterion=From signal port p  InitialConditionsOpt=on
  toChannel : PMIOPort  Port=1  Side=Right
  fromMHS : PMIOPort  Port=2  Side=Left
  toMHS : PMIOPort  Port=3  Side=Right
  wires:
  RoutingControlBehavior/1(route) -> route2Channel1/1
  Constant/1 -> RoutingControlBehavior/2(channel)
  Get Attribute/1 -> RoutingControlBehavior/1(entityChannel)
  serverAvailable/1 -> RoutingControlBehavior/3(serverAvailable)
  connections:
  route2Channel1/RConn2 -- toMHS/RConn1
  Get Attribute/RConn1 -- Single Server1/LConn1
  fromMHS/RConn1 -- Get Attribute/LConn1
  toChannel/RConn1 -- route2Channel1/RConn1
  Single Server1/RConn1 -- route2Channel1/LConn1

== system UberSpurs/spur2WorkCell/route2Channel16 ==
  serverAvailable : Inport
  Constant : Constant  Value=16
  Get Attribute : GetAttribute  AttributeName=Channel  EvaluatedDefaultAttributeValue={ []}
      settings: OutputPortMap=o1
  RoutingControlBehavior : Stateflow chart  TreatAsAtomicUnit=on
  Single Server1 : SingleServer  ServiceTime=0
  route2Channel1 : OutputSwitch  NumberOutputPorts=2  SwitchingCriterion=From signal port p  InitialConditionsOpt=on
  toChannel : PMIOPort  Port=1  Side=Right
  fromMHS : PMIOPort  Port=2  Side=Left
  toMHS : PMIOPort  Port=3  Side=Right
  wires:
  RoutingControlBehavior/1(route) -> route2Channel1/1
  Constant/1 -> RoutingControlBehavior/2(channel)
  Get Attribute/1 -> RoutingControlBehavior/1(entityChannel)
  serverAvailable/1 -> RoutingControlBehavior/3(serverAvailable)
  connections:
  route2Channel1/RConn2 -- toMHS/RConn1
  Get Attribute/RConn1 -- Single Server1/LConn1
  fromMHS/RConn1 -- Get Attribute/LConn1
  toChannel/RConn1 -- route2Channel1/RConn1
  Single Server1/RConn1 -- route2Channel1/LConn1

== system UberSpurs/spur2WorkCell/route2Channel17 ==
  serverAvailable : Inport
  Constant : Constant  Value=17
  Get Attribute : GetAttribute  AttributeName=Channel  EvaluatedDefaultAttributeValue={ []}
      settings: OutputPortMap=o1
  RoutingControlBehavior : Stateflow chart  TreatAsAtomicUnit=on
  Single Server1 : SingleServer  ServiceTime=0
  route2Channel1 : OutputSwitch  NumberOutputPorts=2  SwitchingCriterion=From signal port p  InitialConditionsOpt=on
  toChannel : PMIOPort  Port=1  Side=Right
  fromMHS : PMIOPort  Port=2  Side=Left
  toMHS : PMIOPort  Port=3  Side=Right
  wires:
  RoutingControlBehavior/1(route) -> route2Channel1/1
  Constant/1 -> RoutingControlBehavior/2(channel)
  Get Attribute/1 -> RoutingControlBehavior/1(entityChannel)
  serverAvailable/1 -> RoutingControlBehavior/3(serverAvailable)
  connections:
  route2Channel1/RConn2 -- toMHS/RConn1
  Get Attribute/RConn1 -- Single Server1/LConn1
  fromMHS/RConn1 -- Get Attribute/LConn1
  toChannel/RConn1 -- route2Channel1/RConn1
  Single Server1/RConn1 -- route2Channel1/LConn1

== system UberSpurs/spur2WorkCell/route2Channel18 ==
  serverAvailable : Inport
  Constant : Constant  Value=18
  Get Attribute : GetAttribute  AttributeName=Channel  EvaluatedDefaultAttributeValue={ []}
      settings: OutputPortMap=o1
  RoutingControlBehavior : Stateflow chart  TreatAsAtomicUnit=on
  Single Server1 : SingleServer  ServiceTime=0
  route2Channel1 : OutputSwitch  NumberOutputPorts=2  SwitchingCriterion=From signal port p  InitialConditionsOpt=on
  toChannel : PMIOPort  Port=1  Side=Right
  fromMHS : PMIOPort  Port=2  Side=Left
  toMHS : PMIOPort  Port=3  Side=Right
  wires:
  RoutingControlBehavior/1(route) -> route2Channel1/1
  Constant/1 -> RoutingControlBehavior/2(channel)
  Get Attribute/1 -> RoutingControlBehavior/1(entityChannel)
  serverAvailable/1 -> RoutingControlBehavior/3(serverAvailable)
  connections:
  route2Channel1/RConn2 -- toMHS/RConn1
  Get Attribute/RConn1 -- Single Server1/LConn1
  fromMHS/RConn1 -- Get Attribute/LConn1
  toChannel/RConn1 -- route2Channel1/RConn1
  Single Server1/RConn1 -- route2Channel1/LConn1

== system UberSpurs/spur2WorkCell/route2Channel2 ==
  serverAvailable : Inport
  Constant : Constant  Value=2
  Get Attribute : GetAttribute  AttributeName=Channel  EvaluatedDefaultAttributeValue={ []}
      settings: OutputPortMap=o1
  RoutingControlBehavior : Stateflow chart  TreatAsAtomicUnit=on
  Single Server1 : SingleServer  ServiceTime=0
  route2Channel1 : OutputSwitch  NumberOutputPorts=2  SwitchingCriterion=From signal port p  InitialConditionsOpt=on
  toChannel : PMIOPort  Port=1  Side=Right
  fromMHS : PMIOPort  Port=2  Side=Left
  toMHS : PMIOPort  Port=3  Side=Right
  wires:
  RoutingControlBehavior/1(route) -> route2Channel1/1
  Constant/1 -> RoutingControlBehavior/2(channel)
  Get Attribute/1 -> RoutingControlBehavior/1(entityChannel)
  serverAvailable/1 -> RoutingControlBehavior/3(serverAvailable)
  connections:
  route2Channel1/RConn2 -- toMHS/RConn1
  Get Attribute/RConn1 -- Single Server1/LConn1
  fromMHS/RConn1 -- Get Attribute/LConn1
  toChannel/RConn1 -- route2Channel1/RConn1
  Single Server1/RConn1 -- route2Channel1/LConn1

== system UberSpurs/spur2WorkCell/route2Channel3 ==
  serverAvailable : Inport
  Constant : Constant  Value=3
  Get Attribute : GetAttribute  AttributeName=Channel  EvaluatedDefaultAttributeValue={ []}
      settings: OutputPortMap=o1
  RoutingControlBehavior : Stateflow chart  TreatAsAtomicUnit=on
  Single Server1 : SingleServer  ServiceTime=0
  route2Channel1 : OutputSwitch  NumberOutputPorts=2  SwitchingCriterion=From signal port p  InitialConditionsOpt=on
  toChannel : PMIOPort  Port=1  Side=Right
  fromMHS : PMIOPort  Port=2  Side=Left
  toMHS : PMIOPort  Port=3  Side=Right
  wires:
  RoutingControlBehavior/1(route) -> route2Channel1/1
  Constant/1 -> RoutingControlBehavior/2(channel)
  Get Attribute/1 -> RoutingControlBehavior/1(entityChannel)
  serverAvailable/1 -> RoutingControlBehavior/3(serverAvailable)
  connections:
  route2Channel1/RConn2 -- toMHS/RConn1
  Get Attribute/RConn1 -- Single Server1/LConn1
  fromMHS/RConn1 -- Get Attribute/LConn1
  toChannel/RConn1 -- route2Channel1/RConn1
  Single Server1/RConn1 -- route2Channel1/LConn1

== system UberSpurs/spur2WorkCell/route2Channel4 ==
  serverAvailable : Inport
  Constant : Constant  Value=4
  Get Attribute : GetAttribute  AttributeName=Channel  EvaluatedDefaultAttributeValue={ []}
      settings: OutputPortMap=o1
  RoutingControlBehavior : Stateflow chart  TreatAsAtomicUnit=on
  Single Server1 : SingleServer  ServiceTime=0
  route2Channel1 : OutputSwitch  NumberOutputPorts=2  SwitchingCriterion=From signal port p  InitialConditionsOpt=on
  toChannel : PMIOPort  Port=1  Side=Right
  fromMHS : PMIOPort  Port=2  Side=Left
  toMHS : PMIOPort  Port=3  Side=Right
  wires:
  RoutingControlBehavior/1(route) -> route2Channel1/1
  Constant/1 -> RoutingControlBehavior/2(channel)
  Get Attribute/1 -> RoutingControlBehavior/1(entityChannel)
  serverAvailable/1 -> RoutingControlBehavior/3(serverAvailable)
  connections:
  route2Channel1/RConn2 -- toMHS/RConn1
  Get Attribute/RConn1 -- Single Server1/LConn1
  fromMHS/RConn1 -- Get Attribute/LConn1
  toChannel/RConn1 -- route2Channel1/RConn1
  Single Server1/RConn1 -- route2Channel1/LConn1
